simulink model "dlyj"  (Simulink 2.20)
settings: Solver=ode45  StartTime=0.0  StopTime=10.0  RelTol=1e-3  AbsTol=1e-6
undefined symbols (not defined in the file): offset
settings Model: ConsistencyChecking=off  RTWPlaceOutputsASAP=off  RTWTemplateMakefile=grt_vc.tmf

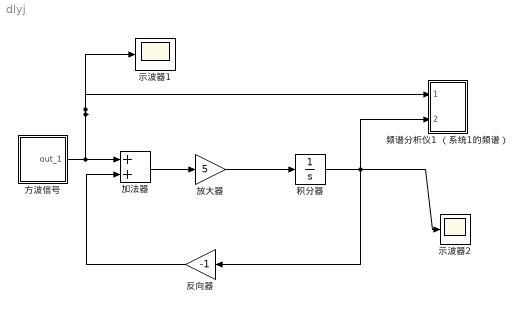
== system dlyj ==
  "   反向器" : Gain  Orientation=left  Gain=-1
  方波信号 : Subsystem  mask(Pulse Generator){@1=20, @2=20, @3=1, @4=1}
      mask prompts: @1 "Pulse period (secs):"; @2 "Pulse width:"; @3 "Pulse height:"; @4 "Pulse start time:"
      mask help: Pulse Generator.
      mask init:
      | Ts=@1; du=@2; ht=@3; stt=@4; ini=ones(length(ht),1); st1=rem(stt,Ts); st2=rem(stt+du,Ts);if(Ts<=1.2*du),ini=zeros(length(ht),1);end;
      mask Help: Pulse generator which ensures pulse\ntransitions are hit. Provides a vector of pulses when the height is entered as a vector.\nUnmask to see how it works.
      mask Display: plot(0,0,100,100,[90,75,75,60,60,35,35,20,20,10],[20,20,80,80,20,20,80,80,20,20])
  放大器 : Gain  Gain=5
  积分器 : Integrator  ExternalReset=none  InitialConditionSource=internal  InitialCondition=0  LimitOutput=off  UpperSaturationLimit=inf  LowerSaturationLimit=-inf  ShowSaturationPort=off  ShowStatePort=off  AbsoluteTolerance=auto
  加法器 : Sum  Inputs=++
  频谱分析仪1 （系统1的频谱） : Subsystem  mask(Spectrum analyzer.){@1=512, @2=1024, @3=100, @4=0.05}
      mask prompts: @1 "Length of buffer:"; @2 "Number of points for fft:"; @3 "Plot after how many points:"; @4 "Sample time:"
      mask help:
      | Spectrum analyser using graph window.
      | Hook input 1 to system input.
      | Hook input 2 to system output.
      mask init:
      | npts=@1; fftpts=@2; HowOften=@3; ts=@4(1); if length(@4) > 1, offset = @4(2), else, offset = 0; end
      mask Help: Hook the system's input to the first port of this block and the system's output to second port. Results are displayed as the frequency response of this system. Use signals with high harmonic content for best results.
      mask Display: plot(0,0,100,100,[11,93,93,11,11],[90,90,40,40,90],[90,80,72,64,55,45,41,36,20],[50,50,52,59,67,75,78,80,80])
  示波器1 : Scope
      settings: TickLabels=on  TimeRange=auto  YMin=-5  YMax=5  SaveToWorkspace=off  SaveName=ScopeData
  示波器2 : Scope
      settings: TickLabels=on  TimeRange=auto  YMin=-5  YMax=5  SaveToWorkspace=off  SaveName=ScopeData
  wires:
  "   反向器"/1 -> 加法器/2
  积分器/1 -> 频谱分析仪1 （系统1的频谱）/2(system output), "   反向器"/1, 示波器2/1
  方波信号/1(out_1) -> 频谱分析仪1 （系统1的频谱）/1(system input), 示波器1/1, 加法器/1
  放大器/1 -> 积分器/1
  加法器/1 -> 放大器/1

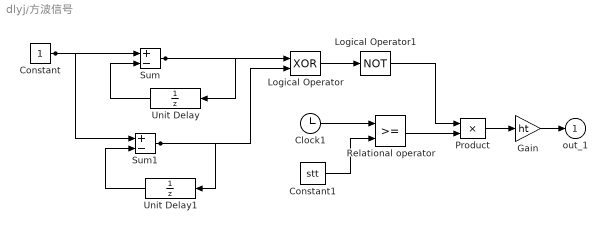
== system dlyj/方波信号 ==
  Clock1 : Clock
  Constant : Constant  Value=1
  Constant1 : Constant  Value=stt
  Gain : Gain  Gain=ht
  Logical Operator : Logic  Operator=XOR  Inputs=2
  Logical Operator1 : Logic  Operator=NOT  Inputs=1
  Product : Product  Inputs=2
  Relational operator : RelationalOperator  Operator=>=
  Sum : Sum  Inputs=+-
  Sum1 : Sum  Inputs=+-
  Unit Delay : UnitDelay  Orientation=left  X0=0  SampleTime=[Ts,st1]
  Unit Delay1 : UnitDelay  Orientation=left  X0=ini  SampleTime=[Ts,st2]
  out_1 : Outport  Port=1
  wires:
  Unit Delay1/1 -> Sum1/2
  Sum1/1 -> Logical Operator/2, Unit Delay1/1
  Constant/1 -> Sum1/1, Sum/1
  Sum/1 -> Logical Operator/1, Unit Delay/1
  Unit Delay/1 -> Sum/2
  Clock1/1 -> Relational operator/1
  Relational operator/1 -> Product/2
  Product/1 -> Gain/1
  Gain/1 -> out_1/1
  Constant1/1 -> Relational operator/2
  Logical Operator/1 -> Logical Operator1/1
  Logical Operator1/1 -> Product/1

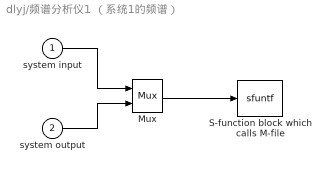
== system dlyj/频谱分析仪1 （系统1的频谱） ==
  system input : Inport  Port=1  PortWidth=-1  SampleTime=-1
  system output : Inport  Port=2  PortWidth=-1  SampleTime=-1
  Mux : Mux  Inputs=2
  S-function block which calls M-file : S-Function  FunctionName=sfuntf  Parameters=fftpts,npts,HowOften,offset,ts,0  PortCounts=[]  SFunctionModules=''
  wires:
  Mux/1 -> S-function block which calls M-file/1
  system input/1 -> Mux/1
  system output/1 -> Mux/2
